simulink model "ALL_PSC_Senarios_Interleaved_Worked_2025_02_11"  (R2024b)
settings: Solver=VariableStepAuto  StartTime=0.0  StopTime=0.05  RelTol=1e-3
values from neighbouring files (symbols this model uses):
  combined_current_new = [combined_current_new, combined_current(minIndex)]    [Temperature_variation.m]
  combined_current_new_Tripple = [0.574 0.574 0.574 0.574 0.574 0.574 0.574 0.574 0.574 0.574 0.574 0.574 ... (17858 elements, 1x17858)]    [combined_current_new_Tripple.mat]
  combined_voltage_new = voltageMin : voltageStep : voltageMax    [Temperature_variation.m]
undefined symbols (not defined in the file or in its folder): combined_voltage_new_Tripple, I_parallel, I_parallel_strong, I_TCT_new, result_Extrapolated_copy, V_parallel, V_TCT_new
libraries: spsSeriesRLCBranchLib x5, spsCurrentMeasurementLib x4, spsMosfetLib x4, spsVoltageMeasurementLib x3, spsControlledCurrentSourceLib x1, spsDiodeLib x1, spsPWMGeneratorDCDCLib x1, sps_lib x1
settings Model: Creator=kimiaahmadi  LastModifiedBy=kimiaahmadi

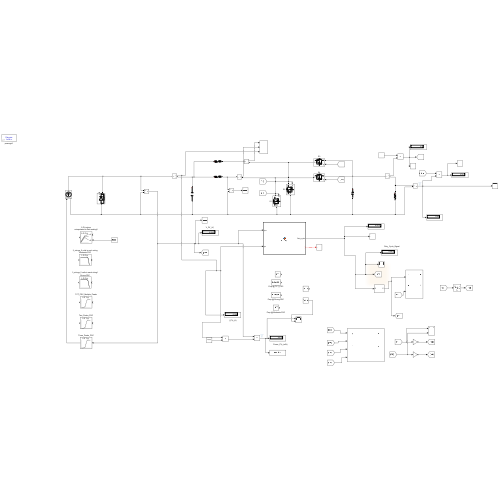
[thumbnail: Simulink's stored preview of the top-level diagram]
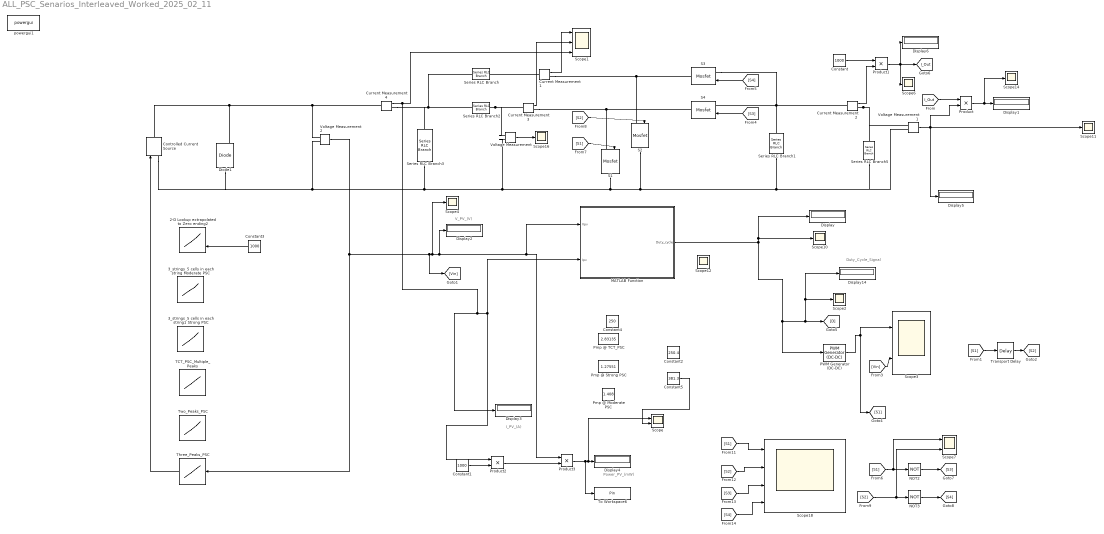
== system ALL_PSC_Senarios_Interleaved_Worked_2025_02_11 ==
  note: Power_PV_(mW)
  note: I_PV_(A)
  note: V_PV_(V)
  note: Duty_Cycle_Signal
  2-D Lookup extrapolated to Zero ending2 : Lookup_n-D  BreakpointsForDimension1=[0:7.058900000000000e-04:0.611]  BreakpointsForDimension2=[1:1000]  Table=[result_Extrapolated_copy].'  ExtrapMethod=Clip  UseLastTableValue=on  InternalRulePriority=Speed  RndMeth=Simplest
      settings: InputPortMap=u0,u1
  3_strings_5 cells in each string Moderate PSC : Lookup_n-D  NumberOfTableDimensions=1  BreakpointsForDimension1=V_parallel  BreakpointsForDimension2=1  BreakpointsForDimension1FirstPoint=0  BreakpointsForDimension1Spacing=0.001714286  BreakpointsForDimension1DataTypeStr=double  UseOneInputPortForAllInputData=on  Table=I_parallel  DiagnosticForOutOfRangeInput=Warning  InternalRulePriority=Speed  RndMeth=Simplest
  3_strings_5 cells in each string1 Strong PSC : Lookup_n-D  NumberOfTableDimensions=1  BreakpointsForDimension1=V_parallel  BreakpointsForDimension2=1  BreakpointsForDimension1FirstPoint=0  BreakpointsForDimension1Spacing=0.001714286  BreakpointsForDimension1DataTypeStr=double  UseOneInputPortForAllInputData=on  Table=I_parallel_strong  DiagnosticForOutOfRangeInput=Warning  InternalRulePriority=Speed  RndMeth=Simplest
  Constant : Constant  Value=1000
  Constant1 : Constant  Value=1000
  Constant2 : Constant  Value=250.4
  Constant3 : Constant  Value=1000
  Constant4 : Constant  Value=250
  Constant5 : Constant  Value=381.3
  Controlled Current Source : spsControlledCurrentSourceLib/Controlled Current Source  Initialize=on  Source_Type=AC  Amplitude=0  Phase=0  Frequency=0  Measurements=None
  Current Measurement{1..4} (4 alike) : spsCurrentMeasurementLib/Current Measurement  PhasorSimulation=off  OutputType=Complex  PSBequivalent=0
  Diode1 : spsDiodeLib/Diode  Ron=0.001  Lon=0  Vf=0  IC=0  UseSnubber=0  Rs=10e5  Cs=250e-9  Measurements=on
  Display{,1..6,14} (8 alike) : Display
  MATLAB Function : MATLAB Function  TreatAsAtomicUnit=on
  NOT2 : Logic  Operator=NOT  IconShape=distinctive  AllPortsSameDT=off  OutDataTypeStr=boolean
  NOT3 : Logic  Operator=NOT  IconShape=distinctive  AllPortsSameDT=off  OutDataTypeStr=boolean
  PWM Generator (DC-DC) : spsPWMGeneratorDCDCLib/PWM Generator (DC-DC)  Fsw=1e6  Ts=0
  Pmp @ Moderate PSC : Constant  Value=1.408
  Pmp @ Strong PSC : Constant  Value=1.27551
  Pmp @ TCT_PSC : Constant  Value=2.83135
  Product{,1..3} (4 alike) : Product
  S{1..4} (4 alike) : spsMosfetLib/Mosfet  Ron=0.1  Lon=0  Rd=0.001  Vfd=0  IC=0  Rs=1e5  Cs=inf  Measurements=off
  Scope : Scope  NumInputPorts=2
  Scope1 : Scope  NumInputPorts=3
  Scope{2,4,6,10..12,14,16} (8 alike) : Scope
  Scope18 : Scope  NumInputPorts=4
  Scope3 : Scope  NumInputPorts=2
  Scope7 : Scope  NumInputPorts=2
  Series RLC Branch : spsSeriesRLCBranchLib/Series RLC Branch  LConnTagsString=__new0  RConnTagsString=__new0  BranchType=RL  Resistance=90e-3  Inductance=2.2e-6  SetiL0=off  InitialCurrent=0  Capacitance=1e-6  Setx0=off  InitialVoltage=0  Measurements=None
  Series RLC Branch1 : spsSeriesRLCBranchLib/Series RLC Branch  LConnTagsString=__new0  RConnTagsString=__new0  BranchType=C  Resistance=0  Inductance=1e-3  SetiL0=off  InitialCurrent=0  Capacitance=10e-6  Setx0=off  InitialVoltage=0  Measurements=None
  Series RLC Branch2 : spsSeriesRLCBranchLib/Series RLC Branch  LConnTagsString=__new0  RConnTagsString=__new0  BranchType=RL  Resistance=90e-3  Inductance=2.2e-6  SetiL0=off  InitialCurrent=0  Capacitance=1e-6  Setx0=off  InitialVoltage=0  Measurements=None
  Series RLC Branch3 : spsSeriesRLCBranchLib/Series RLC Branch  LConnTagsString=__new0  RConnTagsString=__new0  BranchType=C  Resistance=1  Inductance=1e-3  SetiL0=off  InitialCurrent=0  Capacitance=9e-6  Setx0=off  InitialVoltage=0  Measurements=None
  Series RLC Branch5 : spsSeriesRLCBranchLib/Series RLC Branch  LConnTagsString=__new0  RConnTagsString=__new0  BranchType=R  Resistance=5  Inductance=2.2e-6  SetiL0=off  InitialCurrent=0  Capacitance=1e-6  Setx0=off  InitialVoltage=0  Measurements=None
  TCT_PSC_Multiple_Peaks : Lookup_n-D  NumberOfTableDimensions=1  BreakpointsForDimension1=V_TCT_new  BreakpointsForDimension2=1  BreakpointsForDimension1FirstPoint=0  BreakpointsForDimension1Spacing=0.001714286  BreakpointsForDimension1DataTypeStr=double  UseOneInputPortForAllInputData=on  Table=I_TCT_new  DiagnosticForOutOfRangeInput=Warning  InternalRulePriority=Speed  RndMeth=Simplest
  Three_Peaks_PSC : Lookup_n-D  NumberOfTableDimensions=1  BreakpointsForDimension1=combined_voltage_new_Tripple  BreakpointsForDimension2=1  BreakpointsForDimension1FirstPoint=0  BreakpointsForDimension1Spacing=0.001714286  BreakpointsForDimension1DataTypeStr=double  UseOneInputPortForAllInputData=on  Table=combined_current_new_Tripple  DiagnosticForOutOfRangeInput=Warning  InternalRulePriority=Speed  RndMeth=Simplest
  To Workspace6 : ToWorkspace  VariableName=Pin  SampleTime=-1
  Transport Delay : TransportDelay  DelayTime=0.5e-6  BufferSize=100
  Two_Peaks_PSC : Lookup_n-D  NumberOfTableDimensions=1  BreakpointsForDimension1=combined_voltage_new  BreakpointsForDimension2=1  BreakpointsForDimension1FirstPoint=0  BreakpointsForDimension1Spacing=0.001714286  BreakpointsForDimension1DataTypeStr=double  UseOneInputPortForAllInputData=on  Table=combined_current_new  DiagnosticForOutOfRangeInput=Warning  InternalRulePriority=Speed  RndMeth=Simplest
  Voltage Measurement : spsVoltageMeasurementLib/Voltage Measurement  PhasorSimulation=off  OutputType=Complex  PSBequivalent=0
  Voltage Measurement1 : spsVoltageMeasurementLib/Voltage Measurement  PhasorSimulation=off  OutputType=Complex  PSBequivalent=0
  Voltage Measurement2 : spsVoltageMeasurementLib/Voltage Measurement  PhasorSimulation=off  OutputType=Complex  PSBequivalent=0
  powergui1 : sps_lib/powergui  Priority=1  SimulationMode=Discrete  SampleTime=1e-8  frequency=60  Iterations=50  frequencyindice=0  Pbase=100e6  ErrMax=1e-4  UnitsV=kV  UnitsW=MW  buscounter=0  FunctionMessages=off  echomessages=off  EnableUseOfTLC=off  CurrentSourceSwitches=off  DisableSnubberDevices=off  DisableRonSwitches=off  DisableVfSwitches=off  DisplayEquations=off  AutomaticDiscreteSolvers=off  SolverType=Tustin/Backward Euler (TBE)  Interpol=off  ExternalGateDelay=off  methode=off  Ts=100  x0status=blocks  SPID=on  SwTol=0  HookPort=off  NonlinearTolerance=1e-4  nMaxIteration=100  ContinueOnMaxIteration=off  RestoreLinks=warning  ResistiveCurrentMeasurement=off  Frange=[0:2:500]  Ylog=off  Xlog=on  ShowGrid=off  save=off  variable=ZData  structure=0  ZoomFFT=off  StartTime=0.0  cycles=1  DisplayStyle=1  fundamental=60  FreqAxis=off  MaxFrequency=1000  frequencyindicesteady=1  RmsSteady=1  display=off
  tag scope: I_Out=global
  wires:
  [S4] -> S3/1
  [I_Out] -> Product/1
  NOT3/1 -> [S4]
  Voltage Measurement/1 -> Scope16/1
  [S1] -> Transport Delay/1
  Product/1 -> Scope14/1, Display1/1
  Transport Delay/1 -> [S2]
  NOT2/1 -> [S3]
  Product1/1 -> Scope6/1, Display6/1, [I_Out]
  Current Measurement2/1 -> Product1/2
  Voltage Measurement1/1 -> Scope11/1, Display5/1, Product/2
  Product3/1 -> To Workspace6/1, Scope/1, Display4/1
  Product2/1 -> Product3/2
  Current Measurement3/1 -> Scope1/2
  [S2] -> Scope7/2, NOT3/1
  ? -> Scope12/1
  [Vin] -> Scope3/2
  Current Measurement4/1 -> Product2/1, MATLAB Function/2(Ipv), Display3/1, Scope1/3
  [S1] -> Scope7/1, NOT2/1
  [S1] -> Scope18/1
  [S2] -> S2/1
  [S3] -> Scope18/3
  PWM Generator (DC-DC)/1 -> [S1], Scope3/1
  [S4] -> Scope18/4
  [S2] -> Scope18/2
  Constant1/1 -> Product2/2
  [S3] -> S4/1
  Constant/1 -> Product1/1
  Voltage Measurement2/1 -> Three_Peaks_PSC/1, [Vin], Scope4/1, Display2/1, Product3/1, MATLAB Function/1(Vpv)
  Current Measurement1/1 -> Scope1/1
  [S1] -> S1/1
  MATLAB Function/1(Duty_cycle) -> Display/1, Scope10/1, Scope2/1, Display14/1, [D], PWM Generator (DC-DC)/1
  Three_Peaks_PSC/1 -> Controlled Current Source/1
  Constant3/1 -> 2-D Lookup extrapolated to Zero ending2/2
  Constant5/1 -> Scope/2
  connections:
  Current Measurement1/RConn1 -- S2/LConn1 -- S3/RConn1
  S2/RConn1 -- Series RLC Branch5/RConn1 -- Voltage Measurement1/LConn2 -- Series RLC Branch1/RConn1 -- S1/RConn1 -- Series RLC Branch3/RConn1 -- Voltage Measurement2/LConn2 -- Diode1/LConn1 -- Controlled Current Source/LConn1 -- Voltage Measurement/LConn2
  Series RLC Branch2/LConn1 -- Current Measurement4/RConn1 -- Series RLC Branch3/LConn1 -- Series RLC Branch/LConn1
  Series RLC Branch2/RConn1 -- Current Measurement3/LConn1 -- Voltage Measurement/LConn1
  Controlled Current Source/RConn1 -- Voltage Measurement2/LConn1 -- Current Measurement4/LConn1 -- Diode1/RConn1
  Current Measurement3/RConn1 -- S1/LConn1 -- S4/RConn1
  Current Measurement2/RConn1 -- Series RLC Branch5/LConn1 -- Voltage Measurement1/LConn1
  Series RLC Branch1/LConn1 -- S3/LConn1 -- Current Measurement2/LConn1 -- S4/LConn1
  Current Measurement1/LConn1 -- Series RLC Branch/RConn1

== matlab function ALL_PSC_Senarios_Interleaved_Worked_2025_02_11/MATLAB Function ==
  data: Vpv input; Duty_cycle output; Ipv input
function Duty_cycle  = PandO(Vpv, Ipv)

    time_temp  = 400;
    step_size  = 0.01;
    Initial    = 1;
    
   
    persistent Pprev Vprev Dprev time_step dpdv delta_P_prev Dprev_init start Duty_cycle_sweep
    
    if isempty(start)  && Initial == 1
        Pprev      = 0; 
        Vprev      = 0;
        Dprev      = 0;
        Dprev_init = 0;
        time_step  = 1;
        dpdv       = 0;
        delta_P_prev = 0;
        start      = 0;  
        Duty_cycle_sweep = 0;
    end
   
    time_step = mod(time_step + 1, time_temp);
 
    if time_step == 0
        if start == 0
            Ppv = Vpv * Ipv;
            if Ppv > Pprev 
                 Dprev_init = Duty_cycle_sweep;
                 Pprev      = Ppv;
                 Vprev      = Vpv;
             end
    
            Duty_cycle_sweep = Duty_cycle_sweep + step_size;

            if Duty_cycle_sweep >= 0.99 
                start = 1;
                Dprev = Dprev_init;

            end
            
        else
            Ppv        = Vpv * Ipv; 
            delta_P    = Ppv - Pprev; 
            delta_V    = Vpv - Vprev;
            dpdv       = (delta_P) / (delta_V + eps); 
    
            if abs(delta_P_prev - delta_P) < 0.00000095
                deltaD = 0.0;
            else
                deltaD     = abs(dpdv) * 0.004; 
                deltaD     = min(deltaD, 0.01);
            end
    
            % **Perturb & Observe Algorithm**
            if Vpv < 0.0
                D = 0.05;
            elseif dpdv > 0
                D = Dprev - deltaD;
            else
                D = Dprev + deltaD;       
            end 
    
            % Constrain Duty Cycle Limits
            D = max(0, min(0.95, D)); 
    
            % Update previous values for next iteration
            Vprev     = Vpv; 
            Pprev     = Ppv; 
            Dprev     = D;
            delta_P_prev = delta_P;
        end
    end
    
     if start == 1
        Duty_cycle = Dprev;
     else
        Duty_cycle = Duty_cycle_sweep;
     end
end
